simulink model "SolarSailOld"  (R2024a)
settings: Solver=VariableStepAuto  StartTime=0.0  StopTime=60*120  RelTol=1e-3
model workspace (MAT data in the model file):
  LocalBodyOffset = [45 0 0]
undefined symbols (not defined in the file): juliandate, magnitude
libraries: aerolibutil x12, matrix_library x8, aerolibconvert2 x4, sharedtransform x4, slpidlib x2, simulink_extras x2, aerolibsatdyn x1, aerolibobsolete x1, aerolibattitudesys x1, simulink x1, vrlib x1
(part 1 of 2)
settings Model: Creator=pierc  LastModifiedBy=Spare

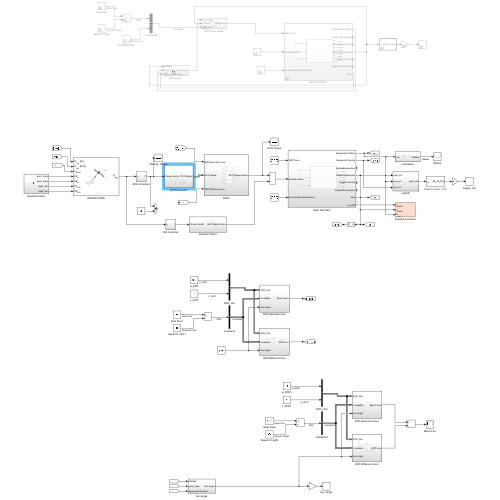
[thumbnail: Simulink's stored preview of the top-level diagram]
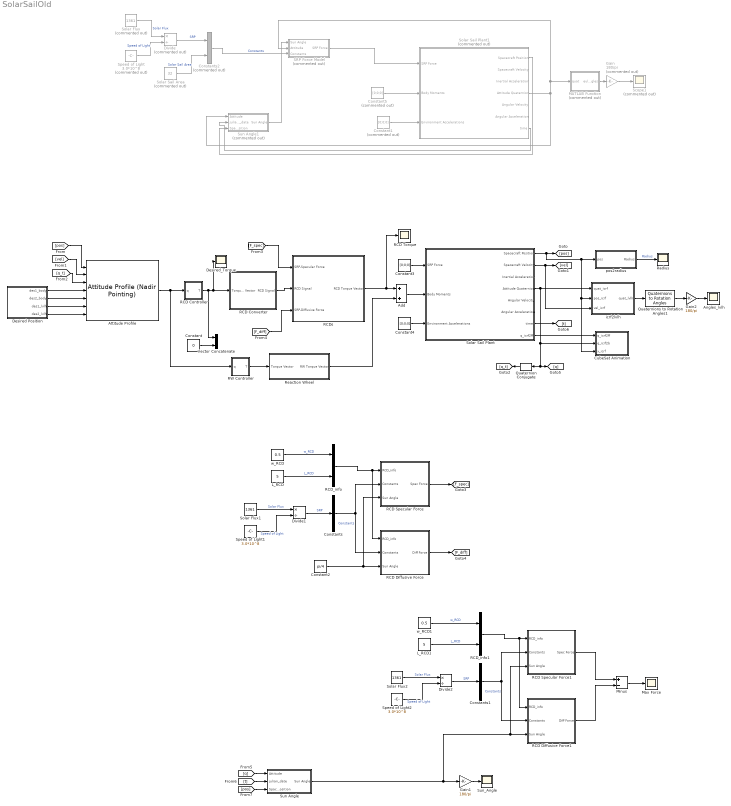
== system SolarSailOld ==
  Add : Sum
  Angles_lvlh : Scope
  "Attitude Profile " : aerolibsatdyn/Attitude Profile (Nadir Pointing)  outputError=on  outputFinalAttitude=off  portFrame=ICRF  pointingMode=Custom  celestialTarget=Sun  tunablePointing=off  primaryAlignmentSrc=Port  primaryAlignment=[0 0 1]  secondaryAlignmentSrc=Port  secondaryAlignment=[1 0 0]  constraintFrame=LVLH  primaryConstraintSrc=Port  primaryConstraint=[1 0 0]  secondaryConstraintSrc=Port  secondaryConstraint=[0 1 0]
  Constant : Constant  Value=0
  Constant1 : Constant  Commented=on  Value=[0;0;0]
  Constant2 : Constant  Value=pi/4
  Constant3 : Constant  Value=[0;0;0]
  Constant4 : Constant  Value=[0;0;0]
  Constant5 : Constant  Commented=on  Value=[0;0;0]
  Constants : BusCreator  Inputs=1
  Constants1 : BusCreator  Inputs=1
  Constants2 : BusCreator  Commented=on  Inputs=2
  CubeSat Animation : Subsystem  mask(Simulink 3D Animation of CubeSat){enableVis=on, startDate=juliandate(2024, 7, 11, 2, 0, 0), visSampleTime=10, cubesatSize=2e5, showAntenna=on, antennaHeight=1e6, antennaHalfAngle=15}
      mask prompts: enableVis "spacecraft:cubesat:AnimEnableVis"; startDate "spacecraft:cubesat:StartDate"; visSampleTime "spacecraft:cubesat:AnimSampleTime"; cubesatSize "spacecraft:cubesat:MdlSize"; showAntenna "spacecraft:cubesat:ShowCone"; antennaHeight "spacecraft:cubesat:ConeHeight"; antennaHalfAngle "spacecraft:cubesat:ConeAngle"
      mask help: spacecraft:cubesat:VisBlockDesc
      settings: OpenFcn=|
      | if ~builtin('license','test','virtual_reality_toolbox')
      |     set_param(gcb, 'enableVis', 'off');
      | end
      | open_system(gcb,'mask');
      mask Callback enableVis:
      | if strcmp(get_param(gcb,'enableVis'), 'on')
      |     [licAvail, ~] = builtin('license','checkout','Virtual_Reality_Toolbox');
      |     if licAvail
      |         enable = repmat({'on'},7,1);
      |         set_param(gcb, 'Commented', 'off');
      |     else
      |         enable = repmat({'off'},7,1);
      |         set_param(gcb, 'Commented', 'on');
      |         set_param(gcb,'enableVis', 'off');
      |     end
      |     clear licAvail
      | else
      |     enable = repmat({'off'},7,1);
      |     set_param(gcb, 'Commented', 'on');
      | end
      | enable{1} = 'on';
      | set_param(gcb,'MaskEnables', enable);
      | clear enable
      mask Callback showAntenna:
      | if strcmp(get_param(gcb, 'enableVis'), 'on')
      |     enable = get_param(gcb,'MaskEnables');
      |     if strcmp(get_param(gcb, 'showAntenna'), 'off')
      |         enable(6:7) = {'off'};
      |     else
      |         enable(6:7) = {'on'};
      |     end
      |     set_param(gcb,'MaskEnables', enable);
      |     clear enable
      | end
      mask DialogControl enableVis Prompt: Enable visualization with Simulink 3D Animation
      mask DialogControl vrOpenBtn Prompt: spacecraft:cubesat:AnimOpenBtn
      mask DialogControl vrOpenBtn Callback:
      | if builtin('license','checkout','Virtual_Reality_Toolbox')
      |     vrmfunc('FnOpen',getSimulinkBlockHandle([gcb '/VR Sink']));
      | end
      mask DialogControl startDate Prompt: Start date [Julian date]:
      mask DialogControl startDate Tooltip: spacecraft:cubesat:StartDateTT
      mask DialogControl visSampleTime Prompt: Animation refresh rate:
      mask DialogControl visSampleTime Tooltip: spacecraft:cubesat:AnimSampleTimeTT
      mask DialogControl cubesatSize Prompt: CubeSat display size [m]:
      mask DialogControl cubesatSize Tooltip: spacecraft:cubesat:MdlSizeTT
      mask DialogControl Container3 Prompt: spacecraft:cubesat:AntennaPropArea
      mask DialogControl showAntenna Prompt: Show antenna cone in animation
      mask DialogControl showAntenna Tooltip: spacecraft:cubesat:ShowConeTT
      mask DialogControl antennaHeight Prompt: Antenna cone height [m]:
      mask DialogControl antennaHeight Tooltip: spacecraft:cubesat:ConeHeightTT
      mask DialogControl antennaHalfAngle Prompt: Antenna cone half angle [deg]:
      mask DialogControl antennaHalfAngle Tooltip: spacecraft:cubesat:ConeAngleTT
      mask Display:
      | port_label('input', 3, 'X_{icrf}','texmode','on')
      | port_label('input', 2, 'q_{icrf2b}','texmode','on')
      | port_label('input', 1, 'q_{icrf2ff}','texmode','on')
  Desired Position : Subsystem
  Desired_Torque : Scope
  Divide : Product  Commented=on  Inputs=*/
  Divide1 : Product  Inputs=*/
  Divide2 : Product  Inputs=*/
  Gain : Gain  Commented=on  Gain=180/pi
  Gain1 : Gain  Gain=180/pi
  Gain2 : Gain  Gain=180/pi
  L_RCD : Constant  Value=5
  L_RCD1 : Constant  Value=5
  MATLAB Function : MATLAB Function  Commented=on  TreatAsAtomicUnit=on
  Max Force : Scope
  Minus : Sum  Inputs=+-
  Quaternion Conjugate : aerolibutil/Quaternion Conjugate
  Quaternions to Rotation Angles1 : sharedtransform/Quaternions to Rotation Angles  rotationOrder=ZYX  aMode=aMode
  RCD Controller : Subsystem
  RCD Converter : Subsystem
  RCD Diffusive Force : Subsystem
  RCD Diffusive Force1 : Subsystem
  RCD Specular Force : Subsystem
  RCD Specular Force1 : Subsystem
  RCD Torque : Scope
  RCD_info : BusCreator  Inputs=2
  RCD_info1 : BusCreator  Inputs=2
  RCDs : Subsystem
  RW Controller : Subsystem
  Radius : Scope
  Reaction Wheel : Subsystem
  SRP Force Model : Subsystem  Commented=on
  Scope1 : Scope  Commented=on
  Solar Flux : Constant  Commented=on  Value=1361
  Solar Flux1 : Constant  Value=1361
  Solar Flux2 : Constant  Value=1361
  Solar Sail Area : Constant  Commented=on  Value=32
  Solar Sail Plant : Subsystem
  Solar Sail Plant1 : Subsystem  Commented=on
  Speed of Light : Constant  Commented=on  Value=3.0*10^8
  Speed of Light1 : Constant  Value=3.0*10^8
  Speed of Light2 : Constant  Value=3.0*10^8
  Sun Angle : Subsystem
  Sun Angle1 : Subsystem  Commented=on
  Sun_Angle : Scope
  Vector Concatenate : Concatenate
  icrf2lvlh : Subsystem
  pos2radius : Subsystem
  w_RCD : Constant  Value=0.5
  w_RCD1 : Constant  Value=0.5
  wires:
  SRP Force Model/1(SRP Force) -> Solar Sail Plant1/1(SRP Force)
  Solar Sail Area/1 -> Constants2/2  "Solar Sail Area"
  Constants2/1 -> SRP Force Model/3(Constants)  "Constants"
  Sun Angle1/1(Sun Angle) -> SRP Force Model/1(Sun Angle)
  Solar Sail Plant1/7(time) -> Sun Angle1/2(julian_date)
  Solar Sail Plant1/1(Spacecraft Position) -> Sun Angle1/3(Spacecraft Position)
  Solar Sail Plant1/4(Attitude Quaternion) -> Sun Angle1/1(Attitude), MATLAB Function/1(quat), SRP Force Model/2(Attitude)
  Constant5/1 -> Solar Sail Plant1/2(Body Moments)
  Constant1/1 -> Solar Sail Plant1/3(Environment Accelerations)
  MATLAB Function/1(eulerAngles) -> Gain/1
  Gain/1 -> Scope1/1
  Solar Sail Plant/1(Spacecraft Position) -> icrf2lvlh/2(pos_icrf), CubeSat Animation/3(x_icrf), pos2radius/1(pos), [pos]
  Solar Sail Plant/4(Attitude Quaternion) -> Quaternion Conjugate/1, [q], CubeSat Animation/2(q_icrf2b), icrf2lvlh/1(quat_icrf)
  Constant3/1 -> Solar Sail Plant/1(SRP Force)
  Constant4/1 -> Solar Sail Plant/3(Environment Accelerations)
  pos2radius/1(Radius) -> Radius/1  "Radius"
  Solar Sail Plant/8(q_icrf2ff) -> CubeSat Animation/1(q_icrf2ff)
  Gain2/1 -> Angles_lvlh/1
  L_RCD/1 -> RCD_info/2  "L_RCD"
  RCD_info/1 -> RCD Diffusive Force/1(RCD_info), RCD Specular Force/1(RCD_info)
  Solar Flux/1 -> Divide/1  "Solar Flux"
  Speed of Light/1 -> Divide/2  "Speed of Light"
  Divide/1 -> Constants2/1  "SRP"
  RCD Controller/1(T) -> Vector Concatenate/1, Desired_Torque/1, RCD Converter/1(Torque Vector)
  [pos] -> "Attitude Profile "/1
  Solar Sail Plant/2(Spacecraft Velocity) -> [vel], icrf2lvlh/3(vel_icrf)
  [vel] -> "Attitude Profile "/2
  Quaternion Conjugate/1 -> [q_t]
  [q_t] -> "Attitude Profile "/3
  Constants/1 -> RCD Specular Force/2(Constants), RCD Diffusive Force/2(Constants)  "Constants"
  Solar Flux1/1 -> Divide1/1  "Solar Flux"
  Speed of Light1/1 -> Divide1/2  "Speed of Light"
  Divide1/1 -> Constants/1  "SRP"
  [F_spec] -> RCDs/1(SRP-Specular Force)
  RCDs/1(RCD Torque Vector) -> Add/1, RCD Torque/1
  RCD Converter/1(RCD Signal) -> RCDs/2(RCD Signal)
  Reaction Wheel/1(RW Torque Vector) -> Add/2
  icrf2lvlh/1(quat_lvlh) -> Quaternions to Rotation Angles1/1
  Quaternions to Rotation Angles1/1 -> Gain2/1
  Desired Position/3(des1_lvlh) -> "Attitude Profile "/6
  Desired Position/4(des2_lvlh) -> "Attitude Profile "/7
  w_RCD/1 -> RCD_info/1  "w_RCD"
  RCD Specular Force/1(Spec Force) -> [F_spec]
  RCD Diffusive Force/1(Diff Force) -> [F_diff]
  [F_diff] -> RCDs/3(SRP-Diffusive Force)
  "Attitude Profile "/1 -> RW Controller/1(q), RCD Controller/1(q)
  Desired Position/1(des1_body) -> "Attitude Profile "/4
  Desired Position/2(des2_body) -> "Attitude Profile "/5
  Add/1 -> Solar Sail Plant/2(Body Moments)
  RW Controller/1(T) -> Reaction Wheel/1(Torque Vector)
  Solar Sail Plant/7(time) -> [t]
  [t] -> Sun Angle/2(julian_date)
  [q] -> Sun Angle/1(Attitude)
  [pos] -> Sun Angle/3(Spacecraft Position)
  Gain1/1 -> Sun_Angle/1
  Constant/1 -> Vector Concatenate/2
  Speed of Light2/1 -> Divide2/2  "Speed of Light"
  w_RCD1/1 -> RCD_info1/1  "w_RCD"
  RCD Specular Force1/1(Spec Force) -> Minus/1
  RCD Diffusive Force1/1(Diff Force) -> Minus/2
  RCD_info1/1 -> RCD Diffusive Force1/1(RCD_info), RCD Specular Force1/1(RCD_info)
  Divide2/1 -> Constants1/1  "SRP"
  Solar Flux2/1 -> Divide2/1  "Solar Flux"
  Constants1/1 -> RCD Specular Force1/2(Constants), RCD Diffusive Force1/2(Constants)  "Constants"
  Sun Angle/1(Sun Angle) -> RCD Specular Force1/3(Sun Angle), RCD Diffusive Force1/3(Sun Angle), Gain1/1
  L_RCD1/1 -> RCD_info1/2  "L_RCD"
  Minus/1 -> Max Force/1
  Constant2/1 -> RCD Specular Force/3(Sun Angle), RCD Diffusive Force/3(Sun Angle)

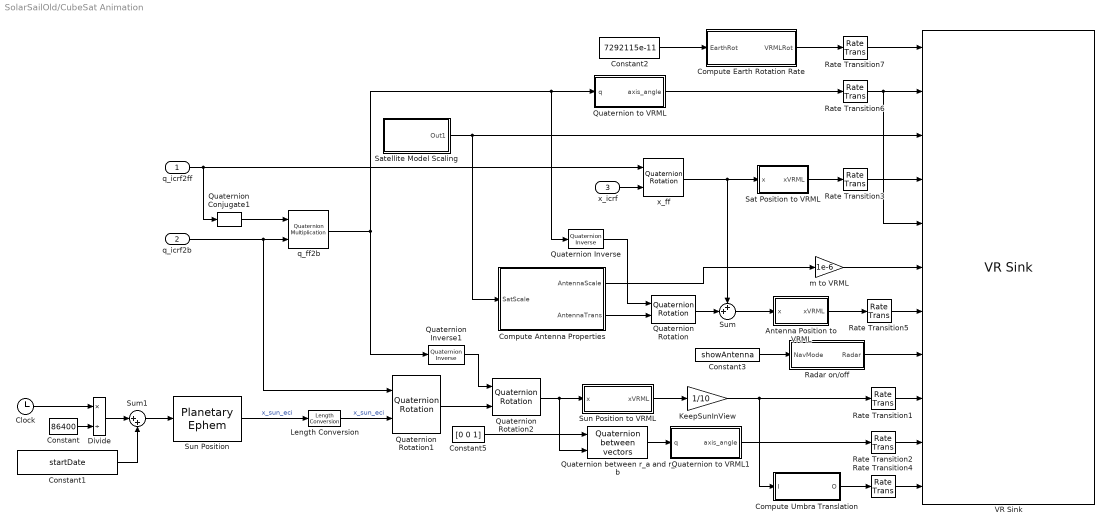
== system SolarSailOld/CubeSat Animation ==
  q_icrf2ff : Inport  PortDimensions=4
  q_icrf2b : Inport  Port=2  PortDimensions=4
  x_icrf : Inport  Port=3  PortDimensions=3
  Antenna Position to VRML : Subsystem
  Clock : Clock
  Compute Antenna Properties : Subsystem
  Compute Earth Rotation Rate : Subsystem
  Compute Umbra Translation : Subsystem
  Constant : Constant  Value=86400
  Constant1 : Constant  Value=startDate  SampleTime=visSampleTime
  Constant2 : Constant  Value=7292115e-11
  Constant3 : Constant  Value=showAntenna
  Constant5 : Constant  Value=[0 0 1]
  Divide : Product  Inputs=*/
  KeepSunInView : Gain  Gain=1/10
  Length Conversion : aerolibconvert2/Length Conversion  IU=km  OU=m
  Quaternion Conjugate1 : aerolibutil/Quaternion Conjugate
  Quaternion Inverse : aerolibutil/Quaternion Inverse
  Quaternion Inverse1 : aerolibutil/Quaternion Inverse
  Quaternion Rotation : aerolibutil/Quaternion Rotation
  Quaternion Rotation1 : aerolibutil/Quaternion Rotation
  Quaternion Rotation2 : aerolibutil/Quaternion Rotation
  Quaternion between r_a and r_b : aerolibattitudesys/Quaternion between vectors
  Quaternion to VRML : Subsystem
  Quaternion to VRML1 : Subsystem
  Radar on/off : Subsystem
  Rate Transition{1..7} (7 alike) : RateTransition
  Sat Position to VRML : Subsystem
  Satellite Model Scaling : Subsystem
  Sum : Sum  Inputs=++|
  Sum1 : Sum  Inputs=|++
  Sun Position : PlanetaryEphem  ephemerisModel=DE421  target=Sun  outputVelocity=off
  Sun Position to VRML : Subsystem
  VR Sink : vrlib/VR Sink  InstantiateOnLoad=on  SampleTime=visSampleTime  ViewEnable=on  RemoteChange=off  RemoteView=off  FieldsWritten=Earth.rotation.4.1.1.double#Satellite.rotation.4.1.1.double#Satellite.scale.3.1.1.double#Satellite.translation.3.1.1.double#AntennaCone.rotation.4.1.1.double#AntennaCone.scale.3.1.1.double#AntennaCone.translation.3.1.1.double#AntennaMaterial.transparency.1.1.1.double#Sun.translation.3.1.1.double#Umbra.rotation.4.1.1.double#Umbra.translation.3.1.1.double  WorldFileName=cubesatAnim.wrl  WorldDescription=CubeSat Orbit Animation  AutoView=off  VideoDimensions=[]  AllowVariableSize=off  FigureProperties="{'Position', 'Name', 'Viewpoint', 'CameraBound', 'CameraDirection', 'CameraPosition', 'CameraUpVector', 'ZoomFactor', 'Antialiasing', 'Headlight', 'Lighting', 'Sound', 'StatusBar', 'Stereo3D', 'Stereo3DCameraOffset', 'Stereo3DHIT', 'ToolBar', 'Textures', 'Transparency', 'Triad', 'Wireframe', 'NavZones', 'NavMode', 'NavSpeed', 'CaptureFileFormat', 'CaptureFileName', 'Record2DCompressMethod', 'Record2DCompressQuality', 'Record2D', 'Record2DFileName', 'Record2DFPS', 'NavPanel'; [1.0000000000000000e+00   7.6000000000000000e+01   1.9200000000000000e+03   9.1300000000000000e+02], 'CubeSat Orbit Animation', 'Satellite-fixed', 'on', [1.8532076975005182e-02   1.5658460164834759e-01  -9.8750612734233556e-01], [5.1717154537575027e-02  -2.3230877286223661e+00  -8.9856200709735745e-01], [-6.2587088021580528e-02   9.8591804959445684e-01   1.5515964991196535e-01], [1.0000000000000000e+00], 'on', 'on', 'on', 'on', 'on', 'off', [1.0000000149011612e-01], [0.0000000000000000e+00], 'on', 'on', 'on', 'none', 'off', 'off', 'examine', 'normal', 'tif', '%f_anim_%n.tif', 'auto', [7.5000000000000000e+01], 'off', '%f_anim_%n.avi', 'auto', 'halfbar'}"
  m to VRML : Gain  Gain=1e-6
  q_ff2b : aerolibutil/Quaternion Multiplication
  x_ff : aerolibutil/Quaternion Rotation
  wires:
  Quaternion to VRML1/1(axis_angle) -> Rate Transition2/1
  Quaternion between r_a and r_b/1 -> Quaternion to VRML1/1(q)
  Constant2/1 -> Compute Earth Rotation Rate/1(EarthRot)
  Compute Antenna Properties/1(AntennaScale) -> m to VRML/1
  Quaternion to VRML/1(axis_angle) -> Rate Transition6/1
  Compute Umbra Translation/1(O) -> Rate Transition4/1
  q_icrf2b/1 -> Quaternion Rotation1/1, q_ff2b/2
  Quaternion Rotation2/1 -> Sun Position to VRML/1(x), Quaternion between r_a and r_b/2
  Constant5/1 -> Quaternion between r_a and r_b/1
  KeepSunInView/1 -> Compute Umbra Translation/1(I), Rate Transition1/1
  Sun Position to VRML/1(xVRML) -> KeepSunInView/1
  Sat Position to VRML/1(xVRML) -> Rate Transition3/1
  Compute Antenna Properties/2(AntennaTrans) -> Quaternion Rotation/2
  Satellite Model Scaling/1(Out1) -> VR Sink/3, Compute Antenna Properties/1(SatScale)
  Constant3/1 -> Radar on/off/1(NavMode)
  q_ff2b/1 -> Quaternion Inverse/1, Quaternion to VRML/1(q), Quaternion Inverse1/1
  Quaternion Rotation1/1 -> Quaternion Rotation2/2
  Compute Earth Rotation Rate/1(VRMLRot) -> Rate Transition7/1
  Antenna Position to VRML/1(xVRML) -> Rate Transition5/1
  Quaternion Inverse/1 -> Quaternion Rotation/1
  x_ff/1 -> Sum/1, Sat Position to VRML/1(x)
  Quaternion Rotation/1 -> Sum/2
  Sum/1 -> Antenna Position to VRML/1(x)
  Quaternion Inverse1/1 -> Quaternion Rotation2/1
  Rate Transition4/1 -> VR Sink/11
  Rate Transition2/1 -> VR Sink/10
  Rate Transition1/1 -> VR Sink/9
  Rate Transition5/1 -> VR Sink/7
  m to VRML/1 -> VR Sink/6
  Rate Transition3/1 -> VR Sink/4
  Rate Transition7/1 -> VR Sink/1
  Rate Transition6/1 -> VR Sink/5, VR Sink/2
  Constant1/1 -> Sum1/2
  Divide/1 -> Sum1/1
  Constant/1 -> Divide/2
  Sun Position/1 -> Length Conversion/1  "x_sun_eci"
  Clock/1 -> Divide/1
  Length Conversion/1 -> Quaternion Rotation1/2  "x_sun_eci"
  Sum1/1 -> Sun Position/1
  Radar on/off/1(Radar) -> VR Sink/8
  Quaternion Conjugate1/1 -> q_ff2b/1
  q_icrf2ff/1 -> Quaternion Conjugate1/1, x_ff/1
  x_icrf/1 -> x_ff/2

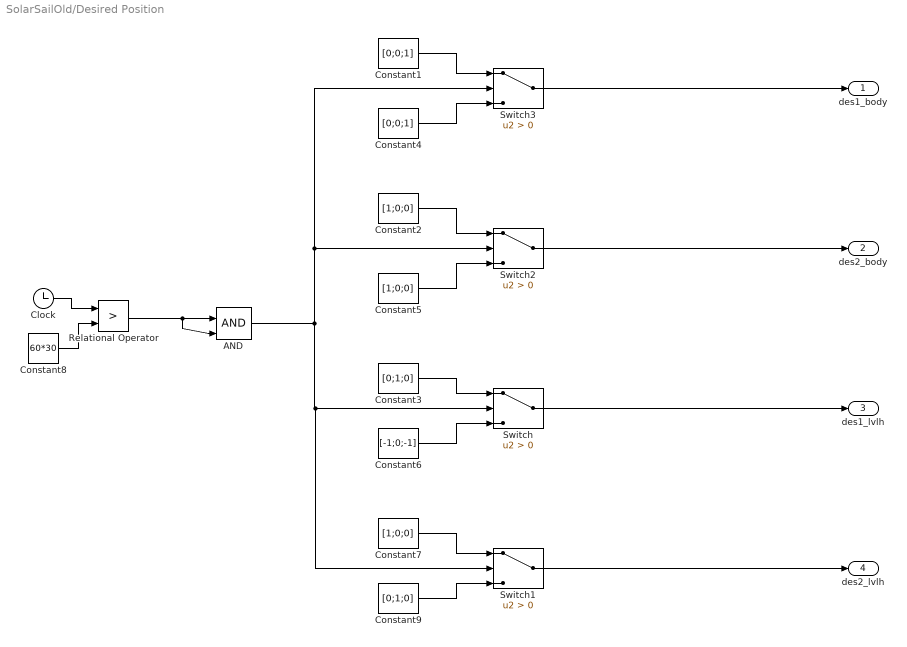
== system SolarSailOld/Desired Position ==
  AND : Logic  IconShape=distinctive  AllPortsSameDT=off  OutDataTypeStr=boolean
  Clock : Clock
  Constant1 : Constant  Value=[0;0;1]
  Constant2 : Constant  Value=[1;0;0]
  Constant3 : Constant  Value=[0;1;0]
  Constant4 : Constant  Value=[0;0;1]
  Constant5 : Constant  Value=[1;0;0]
  Constant6 : Constant  Value=[-1;0;-1]
  Constant7 : Constant  Value=[1;0;0]
  Constant8 : Constant  Value=60*30
  Constant9 : Constant  Value=[0;1;0]
  Relational Operator : RelationalOperator  Operator=>  OutDataTypeStr=boolean  RndMeth=Simplest  InputSameDT=off
  Switch{,1..3} (4 alike) : Switch  Criteria=u2 > Threshold  SaturateOnIntegerOverflow=off  InputSameDT=off
  des1_body : Outport
  des2_body : Outport  Port=2
  des1_lvlh : Outport  Port=3
  des2_lvlh : Outport  Port=4
  wires:
  Constant8/1 -> Relational Operator/2
  Constant6/1 -> Switch/3
  Clock/1 -> Relational Operator/1
  Constant9/1 -> Switch1/3
  Constant4/1 -> Switch3/3
  Constant5/1 -> Switch2/3
  Switch3/1 -> des1_body/1
  Switch2/1 -> des2_body/1
  Switch/1 -> des1_lvlh/1
  Switch1/1 -> des2_lvlh/1
  Constant1/1 -> Switch3/1
  Constant2/1 -> Switch2/1
  Constant7/1 -> Switch1/1
  Constant3/1 -> Switch/1
  AND/1 -> Switch1/2, Switch/2, Switch3/2, Switch2/2
  Relational Operator/1 -> AND/2, AND/1

== system SolarSailOld/RCD Controller ==
  q : Inport
  Demo Controller : slpidlib/PID Controller  Controller=PID  Form=Parallel  TimeDomain=Discrete-time  UseExternalTs=off  SampleTime=-1  IntegratorMethod=Trapezoidal  FilterMethod=Trapezoidal  ControllerParametersSource=internal  P=.0000022  I=0  UseKiTs=off  D=.0015  UseExternalDerivativeSource=off  N=1  UseFilter=off  TunerSelectOption=Transfer Function Based (PID Tuner App)  InitialConditionSource=internal  InitialConditionForIntegrator=0  InitialConditionForFilter=0  DifferentiatorICPrevScaledInput=0  ExternalReset=none  TrackingMode=off  Kt=1  LimitOutput=on  SatLimitsSource=internal  UpperSaturationLimit=0.008  LowerSaturationLimit=-0.008  LinearizeAsGain=on  AntiWindupMode=none  Kb=1  LimitIntegrator=off  UpperIntegratorSaturationLimit=inf  LowerIntegratorSaturationLimit=-inf  POutMin=[]  POutMax=[]  IOutMin=[]  IOutMax=[]  DOutMin=[]  DOutMax=[]  NOutMin=[]  NOutMax=[]  SumOutMin=[]  SumOutMax=[]  SaturationOutMin=[]  SaturationOutMax=[]  PParamMin=[]  PParamMax=[]  IParamMin=[]  IParamMax=[]  DParamMin=[]  DParamMax=[]  NParamMin=[]  NParamMax=[]  KbParamMin=[]  KbParamMax=[]  KtParamMin=[]  KtParamMax=[]  KbOutMin=[]  KbOutMax=[]  KtOutMin=[]  KtOutMax=[]  IntegratorOutMin=[]  IntegratorOutMax=[]  FilterOutMin=[]  FilterOutMax=[]  SumI1OutMin=[]  SumI1OutMax=[]  SumI2OutMin=[]  SumI2OutMax=[]  SumI3OutMin=[]  SumI3OutMax=[]  SumI4OutMin=[]  SumI4OutMax=[]  SumDOutMin=[]  SumDOutMax=[]  DifferentiatorOutMin=[]  DifferentiatorOutMax=[]  FilterDiffOutCoefMin=[]  FilterDiffOutCoefMax=[]  ReciprocalOutMin=[]  ReciprocalOutMax=[]  SumDenOutMin=[]  SumDenOutMax=[]  SumNumOutMin=[]  SumNumOutMax=[]  DivideOutMin=[]  DivideOutMax=[]  UdiffTsProdOutMin=[]  UdiffTsProdOutMax=[]  NTsProdOutMin=[]  NTsProdOutMax=[]  UintegralTsProdOutMin=[]  UintegralTsProdOutMax=[]  UngainTsProdOutMin=[]  UngainTsProdOutMax=[]  ClampingZeroOutDataTypeStr=Inherit: Inherit via back propagation  ClampingZeroOutMin=[]  ClampingZeroOutMax=[]  FilterDenConstantOutDataTypeStr=Inherit: Inherit via back propagation  FilterDenConstantOutMin=[]  FilterDenConstantOutMax=[]  PCopyOutDataTypeStr=Inherit: Inherit via back propagation  PCopyOutMin=[]  PCopyOutMax=[]  NCopyOutDataTypeStr=Inherit: Inherit via back propagation  NCopyOutMin=[]  NCopyOutMax=[]  IntegratorContinuousStateAttributes=''  IntegratorStateMustResolveToSignalObject=off  IntegratorRTWStateStorageClass=Auto  FilterContinuousStateAttributes=''  FilterStateMustResolveToSignalObject=off  FilterRTWStateStorageClass=Auto  ParallelPVariant=InternalParameters  IdealPVariant=Disabled  IVariant=InternalParameters  DVariant=InternalParameters  IntegratorVariant=Discrete  SatVariant=Enabled  AWVariant=Passthrough  PCopyVariant=Disabled  TRVariant=Disabled  FdbkBlocksVariant=Forward  IdealPFdbkVariant=Disabled  SatFdbkVariant=Disabled  DerivativeFilterVariant=Differentiator  NVariant=Passthrough  NCopyVariant=Disabled_SignalSpec  FilterICVariant=InternalICsDifferentiator  IntegratorICVariant=InternalICs  ExternalResetVariant=Disabled  TRSumVariant=Passthrough  SumFdbkVariant=Disabled  SumVariant=Sum_PID  TsampFilterVariant=InternalTs  TsampNgainVariant=Passthrough  TsampIntegralVariant=Disabled_SignalSpec  ExternalSaturationOutDataTypeStr=Inherit: Same as second input  DerivativeSourceVariant=ErrorSignal
  Quaternions to Rotation Angles : sharedtransform/Quaternions to Rotation Angles  rotationOrder=XYZ  aMode=aMode
  Selector : Selector  InputPortWidth=3  IndexOptions=Index vector (dialog)  Indices=[1;2]  OutputSizes=1
  T : Outport
  wires:
  q/1 -> Quaternions to Rotation Angles/1
  Demo Controller/1 -> T/1
  Selector/1 -> Demo Controller/1
  Quaternions to Rotation Angles/1 -> Selector/1

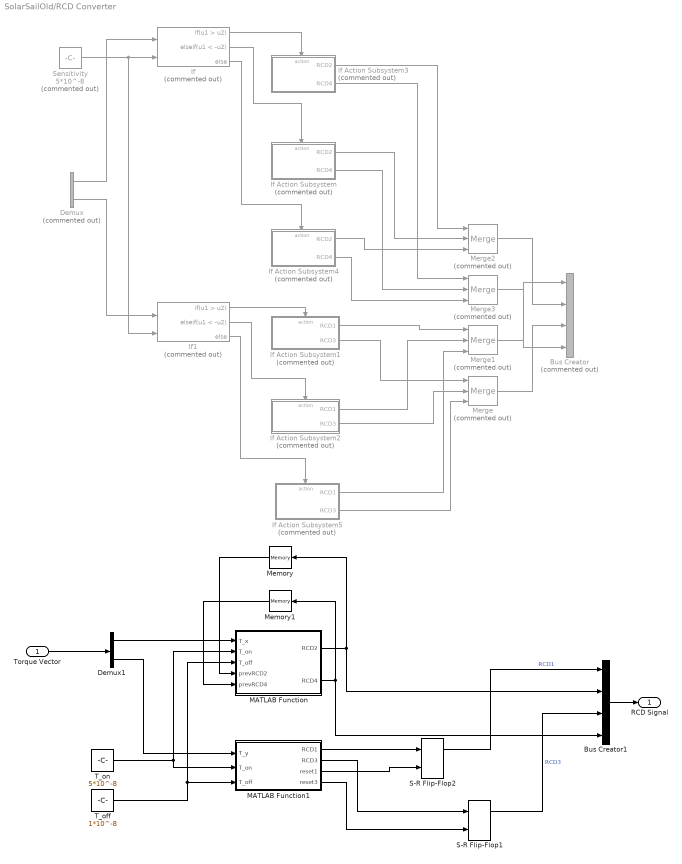
== system SolarSailOld/RCD Converter ==
  Torque Vector : Inport
  Bus Creator : BusCreator  Commented=on  Inputs=4
  Bus Creator1 : BusCreator  Inputs=4
  Demux : Demux  Commented=on  Outputs=2
  Demux1 : Demux  Outputs=2
  If : If  Commented=on  NumInputs=2  IfExpression=u1 > u2  ElseIfExpressions=u1 < -u2
  If Action Subsystem : Subsystem  Commented=on  TreatAsAtomicUnit=on
  If Action Subsystem1 : Subsystem  Commented=on  TreatAsAtomicUnit=on
  If Action Subsystem2 : Subsystem  Commented=on  TreatAsAtomicUnit=on
  If Action Subsystem3 : Subsystem  Commented=on  TreatAsAtomicUnit=on
  If Action Subsystem4 : Subsystem  Commented=on  TreatAsAtomicUnit=on
  If Action Subsystem5 : Subsystem  Commented=on  TreatAsAtomicUnit=on
  If1 : If  Commented=on  NumInputs=2  IfExpression=u1 > u2  ElseIfExpressions=u1 < -u2
  MATLAB Function : MATLAB Function  TreatAsAtomicUnit=on
  MATLAB Function1 : MATLAB Function  TreatAsAtomicUnit=on
  Memory : Memory
  Memory1 : Memory
  Merge{,1..3} (4 alike) : Merge  Commented=on  Inputs=3
  S-R Flip-Flop1 : simulink_extras/Flip Flops/S-R Flip-Flop  initial_condition=0
  S-R Flip-Flop2 : simulink_extras/Flip Flops/S-R Flip-Flop  initial_condition=0
  Sensitivity : Constant  Commented=on  Value=5*10^-8
  T_off : Constant  Value=1*10^-8
  T_on : Constant  Value=5*10^-8
  RCD Signal : Outport
  wires:
  If/1 -> If Action Subsystem3/Action
  If1/1 -> If Action Subsystem1/Action
  If/2 -> If Action Subsystem/Action
  Demux/2 -> If1/1
  Demux/1 -> If/1
  If1/2 -> If Action Subsystem2/Action
  If Action Subsystem1/2(RCD3) -> Merge/1
  Merge/1 -> Bus Creator/3
  If Action Subsystem2/2(RCD3) -> Merge/2
  If Action Subsystem1/1(RCD1) -> Merge1/1
  If Action Subsystem2/1(RCD1) -> Merge1/2
  Merge1/1 -> Bus Creator/1
  Merge2/1 -> Bus Creator/2
  Merge3/1 -> Bus Creator/4
  If Action Subsystem/2(RCD4) -> Merge3/2
  If Action Subsystem/1(RCD2) -> Merge2/2
  If Action Subsystem3/2(RCD4) -> Merge3/1
  If Action Subsystem3/1(RCD2) -> Merge2/1
  Sensitivity/1 -> If/2, If1/2
  If/3 -> If Action Subsystem4/Action
  If Action Subsystem4/2(RCD4) -> Merge3/3
  If Action Subsystem4/1(RCD2) -> Merge2/3
  If1/3 -> If Action Subsystem5/Action
  If Action Subsystem5/1(RCD1) -> Merge1/3
  If Action Subsystem5/2(RCD3) -> Merge/3
  T_on/1 -> MATLAB Function/2(T_on), MATLAB Function1/2(T_on)
  T_off/1 -> MATLAB Function/3(T_off), MATLAB Function1/3(T_off)
  Torque Vector/1 -> Demux1/1
  Demux1/1 -> MATLAB Function/1(T_x)
  Demux1/2 -> MATLAB Function1/1(T_y)
  Bus Creator1/1 -> RCD Signal/1
  MATLAB Function/1(RCD2) -> Memory/1, Bus Creator1/2
  MATLAB Function/2(RCD4) -> Memory1/1, Bus Creator1/4
  Memory/1 -> MATLAB Function/4(prevRCD2)
  Memory1/1 -> MATLAB Function/5(prevRCD4)
  MATLAB Function1/1(RCD1) -> S-R Flip-Flop2/1
  MATLAB Function1/3(reset1) -> S-R Flip-Flop2/2
  MATLAB Function1/2(RCD3) -> S-R Flip-Flop1/1
  MATLAB Function1/4(reset3) -> S-R Flip-Flop1/2
  S-R Flip-Flop1/1 -> Bus Creator1/3  "RCD3"
  S-R Flip-Flop2/1 -> Bus Creator1/1  "RCD1"

== system SolarSailOld/RCD Diffusive Force ==
  Bus Element In : Inport  PortName=RCD_info  Element=w_RCD
  BusElementIn1 : Inport  PortName=RCD_info  Element=L_RCD
  Bus Element In1 : Inport  Port=2  PortName=Constants  Element=SRP
  Sun Angle : Inport  Port=3
  Add : Sum
  Cos : Trigonometry  Operator=cos
  F_normal : Subsystem
  F_sun : Subsystem
  Product : Product
  Product1 : Product
  Diff Force : Outport
  wires:
  BusElementIn1/1 -> Product/1
  Bus Element In/1 -> Product/2
  Sun Angle/1 -> Cos/1, F_sun/3(sun anlge), F_normal/3(sun anlge)
  Bus Element In1/1 -> F_sun/1(SRP), F_normal/1(SRP)
  Product/1 -> F_sun/2(area), F_normal/2(area)  "area"
  F_sun/1(F_sun) -> Product1/1
  Cos/1 -> Product1/2
  Add/1 -> Diff Force/1
  F_normal/1(F_normal) -> Add/1
  Product1/1 -> Add/2

== system SolarSailOld/RCD Diffusive Force1 ==
  Bus Element In : Inport  PortName=RCD_info  Element=w_RCD
  BusElementIn1 : Inport  PortName=RCD_info  Element=L_RCD
  Bus Element In1 : Inport  Port=2  PortName=Constants  Element=SRP
  Sun Angle : Inport  Port=3
  Add : Sum
  Cos : Trigonometry  Operator=cos
  F_normal : Subsystem
  F_sun : Subsystem
  Product : Product
  Product1 : Product
  Diff Force : Outport
  wires:
  BusElementIn1/1 -> Product/1
  Bus Element In/1 -> Product/2
  Sun Angle/1 -> Cos/1, F_sun/3(sun anlge), F_normal/3(sun anlge)
  Bus Element In1/1 -> F_sun/1(SRP), F_normal/1(SRP)
  Product/1 -> F_sun/2(area), F_normal/2(area)  "area"
  F_sun/1(F_sun) -> Product1/1
  Cos/1 -> Product1/2
  Add/1 -> Diff Force/1
  F_normal/1(F_normal) -> Add/1
  Product1/1 -> Add/2

== system SolarSailOld/RCD Specular Force ==
  Bus Element In : Inport  PortName=RCD_info  Element=w_RCD
  BusElementIn1 : Inport  PortName=RCD_info  Element=L_RCD
  Bus Element In1 : Inport  Port=2  PortName=Constants  Element=SRP
  Sun Angle : Inport  Port=3
  Cos : Trigonometry  Operator=cos
  Gain : Gain  Gain=2
  Product : Product
  Product1 : Product  Inputs=3
  Square : Math  Operator=square
  Spec Force : Outport
  wires:
  BusElementIn1/1 -> Product/1
  Bus Element In/1 -> Product/2
  Square/1 -> Product1/3
  Bus Element In1/1 -> Product1/1
  Gain/1 -> Spec Force/1
  Sun Angle/1 -> Cos/1
  Product1/1 -> Gain/1
  Cos/1 -> Square/1
  Product/1 -> Product1/2  "area"

== system SolarSailOld/RCD Specular Force1 ==
  Bus Element In : Inport  PortName=RCD_info  Element=w_RCD
  BusElementIn1 : Inport  PortName=RCD_info  Element=L_RCD
  Bus Element In1 : Inport  Port=2  PortName=Constants  Element=SRP
  Sun Angle : Inport  Port=3
  Cos : Trigonometry  Operator=cos
  Gain : Gain  Gain=2
  Product : Product
  Product1 : Product  Inputs=3
  Square : Math  Operator=square
  Spec Force : Outport
  wires:
  BusElementIn1/1 -> Product/1
  Bus Element In/1 -> Product/2
  Square/1 -> Product1/3
  Bus Element In1/1 -> Product1/1
  Gain/1 -> Spec Force/1
  Sun Angle/1 -> Cos/1
  Product1/1 -> Gain/1
  Cos/1 -> Square/1
  Product/1 -> Product1/2  "area"

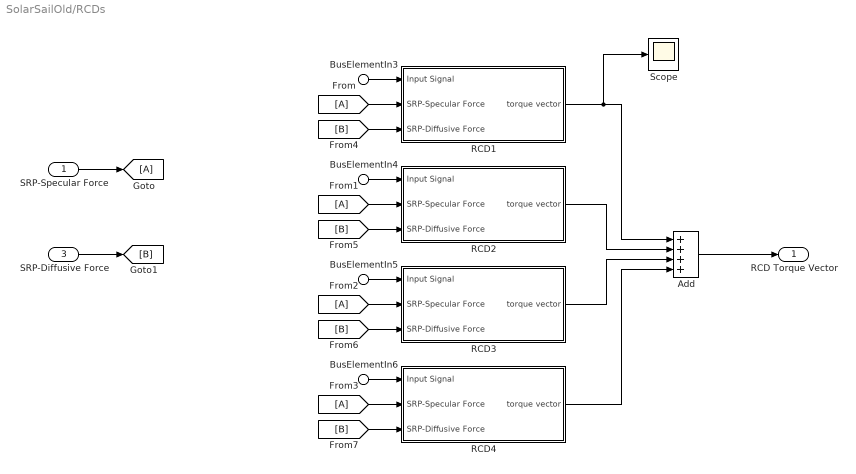
== system SolarSailOld/RCDs ==
  SRP-Specular Force : Inport
  BusElementIn3 : Inport  Port=2  PortName=RCD Signal  Element=RCD1
  BusElementIn4 : Inport  Port=2  PortName=RCD Signal  Element=RCD2
  BusElementIn5 : Inport  Port=2  PortName=RCD Signal  Element=RCD3
  BusElementIn6 : Inport  Port=2  PortName=RCD Signal  Element=RCD4
  SRP-Diffusive Force : Inport  Port=3
  Add : Sum  Inputs=++++
  From{,1..3} (4 alike) : From
  Goto : Goto
  RCD1 : Subsystem
  RCD2 : Subsystem
  RCD3 : Subsystem
  RCD4 : Subsystem
  Scope : Scope
  RCD Torque Vector : Outport
  wires:
  RCD2/1(torque vector) -> Add/2
  RCD1/1(torque vector) -> Scope/1, Add/1
  RCD4/1(torque vector) -> Add/4
  RCD3/1(torque vector) -> Add/3
  Add/1 -> RCD Torque Vector/1
  BusElementIn3/1 -> RCD1/1(Input Signal)
  BusElementIn4/1 -> RCD2/1(Input Signal)
  BusElementIn5/1 -> RCD3/1(Input Signal)
  SRP-Specular Force/1 -> Goto/1
  From/1 -> RCD1/2(SRP-Specular Force)
  From1/1 -> RCD2/2(SRP-Specular Force)
  From2/1 -> RCD3/2(SRP-Specular Force)
  From3/1 -> RCD4/2(SRP-Specular Force)
  [B] -> RCD1/3(SRP-Diffusive Force)
  [B] -> RCD2/3(SRP-Diffusive Force)
  [B] -> RCD3/3(SRP-Diffusive Force)
  [B] -> RCD4/3(SRP-Diffusive Force)
  SRP-Diffusive Force/1 -> [B]
  BusElementIn6/1 -> RCD4/1(Input Signal)

== system SolarSailOld/RW Controller ==
  q : Inport
  Demo Controller : slpidlib/PID Controller  Controller=PD  Form=Parallel  TimeDomain=Discrete-time  UseExternalTs=off  SampleTime=-1  IntegratorMethod=Trapezoidal  FilterMethod=Trapezoidal  ControllerParametersSource=internal  P=.000055  I=0  UseKiTs=off  D=.017  UseExternalDerivativeSource=off  N=1  UseFilter=off  TunerSelectOption=Transfer Function Based (PID Tuner App)  InitialConditionSource=internal  InitialConditionForIntegrator=0  InitialConditionForFilter=0  DifferentiatorICPrevScaledInput=0  ExternalReset=none  TrackingMode=off  Kt=1  LimitOutput=on  SatLimitsSource=internal  UpperSaturationLimit=0.008  LowerSaturationLimit=-0.008  LinearizeAsGain=on  AntiWindupMode=none  Kb=1  LimitIntegrator=off  UpperIntegratorSaturationLimit=inf  LowerIntegratorSaturationLimit=-inf  POutMin=[]  POutMax=[]  IOutMin=[]  IOutMax=[]  DOutMin=[]  DOutMax=[]  NOutMin=[]  NOutMax=[]  SumOutMin=[]  SumOutMax=[]  SaturationOutMin=[]  SaturationOutMax=[]  PParamMin=[]  PParamMax=[]  IParamMin=[]  IParamMax=[]  DParamMin=[]  DParamMax=[]  NParamMin=[]  NParamMax=[]  KbParamMin=[]  KbParamMax=[]  KtParamMin=[]  KtParamMax=[]  KbOutMin=[]  KbOutMax=[]  KtOutMin=[]  KtOutMax=[]  IntegratorOutMin=[]  IntegratorOutMax=[]  FilterOutMin=[]  FilterOutMax=[]  SumI1OutMin=[]  SumI1OutMax=[]  SumI2OutMin=[]  SumI2OutMax=[]  SumI3OutMin=[]  SumI3OutMax=[]  SumI4OutMin=[]  SumI4OutMax=[]  SumDOutMin=[]  SumDOutMax=[]  DifferentiatorOutMin=[]  DifferentiatorOutMax=[]  FilterDiffOutCoefMin=[]  FilterDiffOutCoefMax=[]  ReciprocalOutMin=[]  ReciprocalOutMax=[]  SumDenOutMin=[]  SumDenOutMax=[]  SumNumOutMin=[]  SumNumOutMax=[]  DivideOutMin=[]  DivideOutMax=[]  UdiffTsProdOutMin=[]  UdiffTsProdOutMax=[]  NTsProdOutMin=[]  NTsProdOutMax=[]  UintegralTsProdOutMin=[]  UintegralTsProdOutMax=[]  UngainTsProdOutMin=[]  UngainTsProdOutMax=[]  ClampingZeroOutDataTypeStr=Inherit: Inherit via back propagation  ClampingZeroOutMin=[]  ClampingZeroOutMax=[]  FilterDenConstantOutDataTypeStr=Inherit: Inherit via back propagation  FilterDenConstantOutMin=[]  FilterDenConstantOutMax=[]  PCopyOutDataTypeStr=Inherit: Inherit via back propagation  PCopyOutMin=[]  PCopyOutMax=[]  NCopyOutDataTypeStr=Inherit: Inherit via back propagation  NCopyOutMin=[]  NCopyOutMax=[]  IntegratorContinuousStateAttributes=''  IntegratorStateMustResolveToSignalObject=off  IntegratorRTWStateStorageClass=Auto  FilterContinuousStateAttributes=''  FilterStateMustResolveToSignalObject=off  FilterRTWStateStorageClass=Auto  ParallelPVariant=InternalParameters  IdealPVariant=Disabled  IVariant=Disabled  DVariant=InternalParameters  IntegratorVariant=Disabled  SatVariant=Enabled  AWVariant=Disabled  PCopyVariant=Disabled  TRVariant=Disabled  FdbkBlocksVariant=Forward  IdealPFdbkVariant=Disabled  SatFdbkVariant=Disabled  DerivativeFilterVariant=Differentiator  NVariant=Passthrough  NCopyVariant=Disabled_SignalSpec  FilterICVariant=InternalICsDifferentiator  IntegratorICVariant=Disabled  ExternalResetVariant=Disabled  TRSumVariant=Passthrough  SumFdbkVariant=Disabled  SumVariant=Sum_PD  TsampFilterVariant=InternalTs  TsampNgainVariant=Passthrough  TsampIntegralVariant=Disabled_SignalSpec  ExternalSaturationOutDataTypeStr=Inherit: Same as second input  DerivativeSourceVariant=ErrorSignal
  Quaternions to Rotation Angles : sharedtransform/Quaternions to Rotation Angles  rotationOrder=XYZ  aMode=aMode
  Selector : Selector  InputPortWidth=3  IndexOptions=Index vector (dialog)  Indices=[3]  OutputSizes=1
  T : Outport
  wires:
  q/1 -> Quaternions to Rotation Angles/1
  Quaternions to Rotation Angles/1 -> Selector/1
  Demo Controller/1 -> T/1
  Selector/1 -> Demo Controller/1

== system SolarSailOld/Reaction Wheel ==
  Torque Vector : Inport
  Constant : Constant  Value=10^-3
  Constant7 : Constant  Value=[0;0]
  Torque Limiter : MATLAB Function  TreatAsAtomicUnit=on
  Vector Concatenate : Concatenate
  RW Torque Vector : Outport
  wires:
  Vector Concatenate/1 -> RW Torque Vector/1
  Constant7/1 -> Vector Concatenate/1
  Constant/1 -> Torque Limiter/2(limit)
  Torque Limiter/1(T) -> Vector Concatenate/2
  Torque Vector/1 -> Torque Limiter/1(desired_T)

== system SolarSailOld/SRP Force Model ==
  Sun Angle : Inport
  Attitude : Inport  Port=2
  BusElementIn : Inport  Port=3  PortName=Constants  Element=SRP
  BusElementIn1 : Inport  Port=3  PortName=Constants  Element=Solar Sail Area
  Multiplication : Subsystem
  Normal : Constant  Value=[0;0;1]
  Product : Product  Multiplication=Matrix(*)
  Product1 : Product
  Quat2RotMat : MATLAB Function  TreatAsAtomicUnit=on
  SRP Force : Outport
  wires:
  Sun Angle/1 -> Multiplication/2(Sun Angle)
  Attitude/1 -> Quat2RotMat/1(quat)
  Product/1 -> Product1/2
  Quat2RotMat/1(rotm) -> Product/1
  Normal/1 -> Product/2
  Multiplication/1(SRP Force) -> Product1/1
  Product1/1 -> SRP Force/1
  BusElementIn/1 -> Multiplication/1(SRP)
  BusElementIn1/1 -> Multiplication/3(Area)

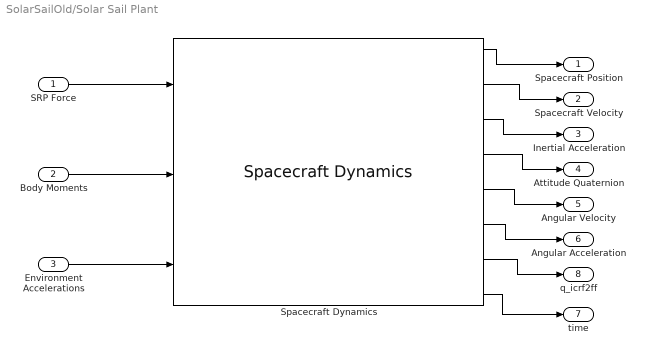
== system SolarSailOld/Solar Sail Plant ==
  SRP Force : Inport
  Body Moments : Inport  Port=2
  Environment Accelerations : Inport  Port=3
  Spacecraft Dynamics : SpacecraftDynamics  accelIn=on  outputAccel=on  startDate=juliandate(2024, 7, 11, 2, 0, 0)  mass=3.0  inertia=[1,0,0;0,1,0;0,0,1]  semiMajorAxis=7078140  eccentricity=0.001  inclination=98.1928  raan=22  argPeriapsis=360  trueAnomaly=0  attitude=[0.719,-0.0985,-0.6633,-0.1827]  outputAngAccel=on  outputTransform=on  ephemerisModel=DE432t  srpArea=32
  Spacecraft Position : Outport
  Spacecraft Velocity : Outport  Port=2
  Inertial Acceleration : Outport  Port=3
  Attitude Quaternion : Outport  Port=4
  Angular Velocity : Outport  Port=5
  Angular Acceleration : Outport  Port=6
  time : Outport  Port=7
  q_icrf2ff : Outport  Port=8
  wires:
  Environment Accelerations/1 -> Spacecraft Dynamics/3
  Body Moments/1 -> Spacecraft Dynamics/2
  SRP Force/1 -> Spacecraft Dynamics/1
  Spacecraft Dynamics/1 -> Spacecraft Position/1
  Spacecraft Dynamics/2 -> Spacecraft Velocity/1
  Spacecraft Dynamics/3 -> Inertial Acceleration/1
  Spacecraft Dynamics/4 -> Attitude Quaternion/1
  Spacecraft Dynamics/5 -> Angular Velocity/1
  Spacecraft Dynamics/6 -> Angular Acceleration/1
  Spacecraft Dynamics/8 -> time/1
  Spacecraft Dynamics/7 -> q_icrf2ff/1

== system SolarSailOld/Solar Sail Plant1 ==
  SRP Force : Inport
  Body Moments : Inport  Port=2
  Environment Accelerations : Inport  Port=3
  Spacecraft Dynamics : SpacecraftDynamics  accelIn=on  accelFrame=Fixed-frame  outportFrame=Fixed-frame  outputAccel=on  mass=3.0  inertia=[344.15, 0, 0; 0, 344.15, 0; 0, 0, 688.24]  semiMajorAxis=7078140  eccentricity=0.001  inclination=98.1928  raan=22  argPeriapsis=360  trueAnomaly=0  attitudeFrame=LVLH  attitude=[0.6533,-0.2706,0.2706,-0.6533]  outputAngAccel=on  ephemerisModel=DE432t  srpArea=32
  Spacecraft Position : Outport
  Spacecraft Velocity : Outport  Port=2
  Inertial Acceleration : Outport  Port=3
  Attitude Quaternion : Outport  Port=4
  Angular Velocity : Outport  Port=5
  Angular Acceleration : Outport  Port=6
  time : Outport  Port=7
  wires:
  Environment Accelerations/1 -> Spacecraft Dynamics/3
  Body Moments/1 -> Spacecraft Dynamics/2
  SRP Force/1 -> Spacecraft Dynamics/1
  Spacecraft Dynamics/1 -> Spacecraft Position/1
  Spacecraft Dynamics/2 -> Spacecraft Velocity/1
  Spacecraft Dynamics/3 -> Inertial Acceleration/1
  Spacecraft Dynamics/4 -> Attitude Quaternion/1
  Spacecraft Dynamics/5 -> Angular Velocity/1
  Spacecraft Dynamics/6 -> Angular Acceleration/1
  Spacecraft Dynamics/7 -> time/1

== system SolarSailOld/Sun Angle ==
  Attitude : Inport
  julian_date : Inport  Port=2
  Spacecraft Position : Inport  Port=3
  MATLAB Function : MATLAB Function  TreatAsAtomicUnit=on
  Math Function : Math  Operator=magnitude^2
  Normal : Constant  Value=[0;0;1]
  Product : Product  Multiplication=Matrix(*)
  Quat2RotMat : MATLAB Function  TreatAsAtomicUnit=on
  Subtract : Sum  Inputs=+-
  sun_position : MATLAB Function  TreatAsAtomicUnit=on
  Sun Angle : Outport
  wires:
  Normal/1 -> Product/2
  Quat2RotMat/1(rotm) -> Product/1
  Product/1 -> MATLAB Function/1(N_icrf)  "N_icrf"
  Attitude/1 -> Quat2RotMat/1(quat)
  Subtract/1 -> MATLAB Function/2(r_satsun)  "r_satsun"
  Spacecraft Position/1 -> Subtract/2  "r_sat"
  sun_position/1(r_sun) -> Subtract/1  "r_sun"
  julian_date/1 -> sun_position/1(julian_date)
  MATLAB Function/1(sunAngle) -> Sun Angle/1

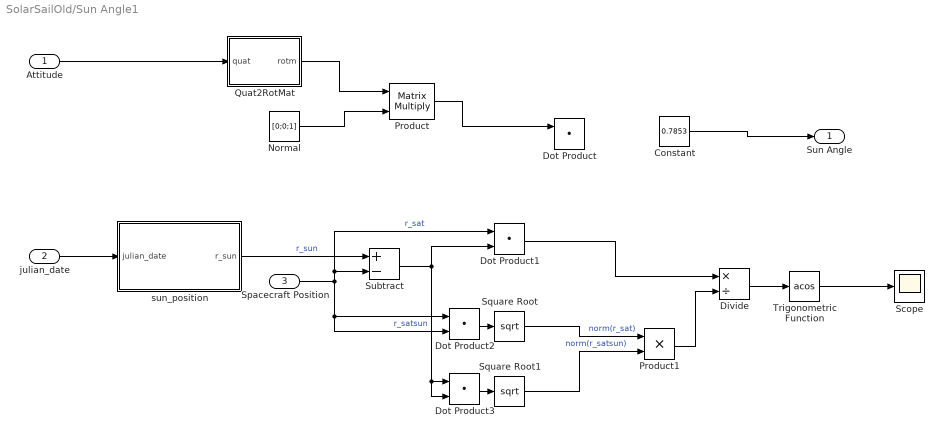
== system SolarSailOld/Sun Angle1 ==
  Attitude : Inport
  julian_date : Inport  Port=2
  Spacecraft Position : Inport  Port=3
  Constant : Constant  Value=0.7853
  Divide : Product  Inputs=*/
  Dot Product{,1..3} (4 alike) : DotProduct  OutDataTypeStr=Inherit: Inherit via internal rule
  Normal : Constant  Value=[0;0;1]
  Product : Product  Multiplication=Matrix(*)
  Product1 : Product
  Quat2RotMat : MATLAB Function  TreatAsAtomicUnit=on
  Scope : Scope
  Square Root : Sqrt
  Square Root1 : Sqrt
  Subtract : Sum  Inputs=+-
  Trigonometric Function : Trigonometry  Operator=acos
  sun_position : MATLAB Function  TreatAsAtomicUnit=on
  Sun Angle : Outport
  wires:
  julian_date/1 -> sun_position/1(julian_date)
  sun_position/1(r_sun) -> Subtract/1  "r_sun"
  Spacecraft Position/1 -> Dot Product1/1, Subtract/2, Dot Product2/2, Dot Product2/1  "r_sat"
  Subtract/1 -> Dot Product3/2, Dot Product3/1, Dot Product1/2  "r_satsun"
  Attitude/1 -> Quat2RotMat/1(quat)
  Product/1 -> Dot Product/1
  Quat2RotMat/1(rotm) -> Product/1
  Normal/1 -> Product/2
  Dot Product2/1 -> Square Root/1
  Dot Product3/1 -> Square Root1/1
  Square Root/1 -> Product1/1  "norm(r_sat)"
  Square Root1/1 -> Product1/2  "norm(r_satsun)"
  Dot Product1/1 -> Divide/1
  Product1/1 -> Divide/2
  Divide/1 -> Trigonometric Function/1
  Trigonometric Function/1 -> Scope/1
  Constant/1 -> Sun Angle/1

== system SolarSailOld/icrf2lvlh ==
  quat_icrf : Inport
  pos_icrf : Inport  Port=2
  vel_icrf : Inport  Port=3
  Direction Cosine Matrix to Quaternions : sharedtransform/Direction Cosine Matrix  to Quaternions  aMode=0  action=Warning  tolerance=eps(4)
      settings: LibrarySourceBlock=|
      | aerolibtransform2/Direction Cosine Matrix
      | to Quaternions
  MATLAB Function : MATLAB Function  TreatAsAtomicUnit=on
  Quaternion Multiplication : aerolibutil/Quaternion Multiplication
  quat_lvlh : Outport
  wires:
  pos_icrf/1 -> MATLAB Function/1(pos)
  vel_icrf/1 -> MATLAB Function/2(vel)
  MATLAB Function/1(DCM) -> Direction Cosine Matrix to Quaternions/1
  quat_icrf/1 -> Quaternion Multiplication/2
  Direction Cosine Matrix to Quaternions/1 -> Quaternion Multiplication/1
  Quaternion Multiplication/1 -> quat_lvlh/1

== system SolarSailOld/pos2radius ==
  pos : Inport
  Dot Product : DotProduct  OutDataTypeStr=Inherit: Inherit via internal rule
  Square Root : Sqrt
  Radius : Outport
  wires:
  pos/1 -> Dot Product/2, Dot Product/1
  Dot Product/1 -> Square Root/1
  Square Root/1 -> Radius/1  "Radius"

== system SolarSailOld/CubeSat Animation/Antenna Position to VRML ==
  x : Inport
  ECEF to VRML : Subsystem
  Length Conversion : aerolibconvert2/Length Conversion  IU=m  OU=km
  km to VRML units : Gain  Gain=1/1000
  xVRML : Outport  VectorParamsAs1DForOutWhenUnconnected=off
  wires:
  Length Conversion/1 -> km to VRML units/1
  km to VRML units/1 -> ECEF to VRML/1(M)
  x/1 -> Length Conversion/1
  ECEF to VRML/1(VR) -> xVRML/1

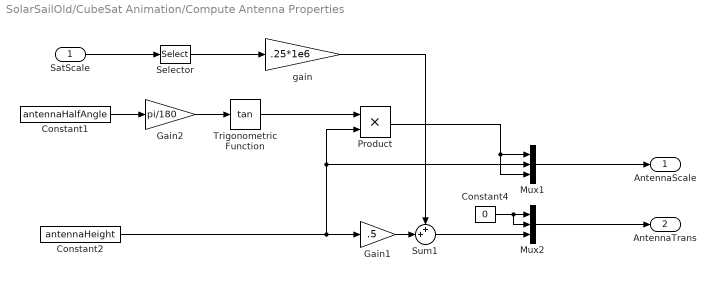
== system SolarSailOld/CubeSat Animation/Compute Antenna Properties ==
  SatScale : Inport
  Constant1 : Constant  Value=antennaHalfAngle
  Constant2 : Constant  Value=antennaHeight
  Constant4 : Constant  Value=0
  Gain1 : Gain  Gain=.5
  Gain2 : Gain  Gain=pi/180
  Mux1 : Mux  Inputs=3
  Mux2 : Mux  Inputs=3
  Product : Product
  Selector : Selector  InputPortWidth=3  IndexOptions=Index vector (dialog)  Indices=1  OutputSizes=1
  Sum1 : Sum  Inputs=++|
  Trigonometric Function : Trigonometry  Operator=tan
  gain : Gain  Gain=.25*1e6
  AntennaScale : Outport  VectorParamsAs1DForOutWhenUnconnected=off
  AntennaTrans : Outport  Port=2  VectorParamsAs1DForOutWhenUnconnected=off
  wires:
  Gain2/1 -> Trigonometric Function/1
  Constant4/1 -> Mux2/1, Mux2/2
  Sum1/1 -> Mux2/3
  Constant2/1 -> Gain1/1, Mux1/2, Product/2
  gain/1 -> Sum1/1
  Constant1/1 -> Gain2/1
  Product/1 -> Mux1/3, Mux1/1
  Gain1/1 -> Sum1/2
  Trigonometric Function/1 -> Product/1
  Mux2/1 -> AntennaTrans/1
  Mux1/1 -> AntennaScale/1
  SatScale/1 -> Selector/1
  Selector/1 -> gain/1

== system SolarSailOld/CubeSat Animation/Compute Earth Rotation Rate ==
  EarthRot : Inport
  Constant : Constant  Value=0
  Constant1 : Constant  Value=0
  Euler Angles to Quaternions : aerolibobsolete/Euler Angles to Quaternions
  Quaternion to VRML : Subsystem
  Sum : Sum  Inputs=|++
  Unit Delay : UnitDelay  SampleTime=-1  HasFrameUpgradeWarning=on
  Vector Concatenate : Concatenate  NumInputs=3
  VRMLRot : Outport  VectorParamsAs1DForOutWhenUnconnected=off
  wires:
  Quaternion to VRML/1(AxisAngle) -> VRMLRot/1
  Euler Angles to Quaternions/1 -> Quaternion to VRML/1(q)
  Vector Concatenate/1 -> Euler Angles to Quaternions/1
  Constant1/1 -> Vector Concatenate/2
  Constant/1 -> Vector Concatenate/1
  Sum/1 -> Unit Delay/1, Vector Concatenate/3
  Unit Delay/1 -> Sum/2
  EarthRot/1 -> Sum/1

== system SolarSailOld/CubeSat Animation/Compute Umbra Translation ==
  I : Inport
  Add : Sum
  ConeHalfLength : Gain  Gain=692
  InvertSunPosECEF : Gain  Gain=-1
  unitVec : Subsystem
  O : Outport  VectorParamsAs1DForOutWhenUnconnected=off
  wires:
  ConeHalfLength/1 -> Add/2
  I/1 -> InvertSunPosECEF/1
  Add/1 -> O/1
  InvertSunPosECEF/1 -> unitVec/1(I), Add/1
  unitVec/1(O) -> ConeHalfLength/1

== system SolarSailOld/CubeSat Animation/Quaternion to VRML ==
  q : Inport
  Demux : Demux
  "Flip 180 deg, rotate 90" : Constant  Value=[0 -.7071 .7071 0]
  Gain : Gain  Gain=2
  Mux : Mux
  Quaternion Multiplication : aerolibutil/Quaternion Multiplication
  Selector : Selector  InputPortWidth=4  IndexOptions=Index vector (dialog)  Indices=[3 4 2 1]  OutputSizes=1
  Trigonometric Function : Trigonometry  Operator=acos
  axis_angle : Outport  VectorParamsAs1DForOutWhenUnconnected=off
  wires:
  Demux/4 -> Mux/4
  Demux/3 -> Mux/3
  Demux/2 -> Mux/2
  Gain/1 -> Mux/1
  Selector/1 -> axis_angle/1
  q/1 -> Quaternion Multiplication/1
  Mux/1 -> Selector/1
  Trigonometric Function/1 -> Gain/1
  Demux/1 -> Trigonometric Function/1
  "Flip 180 deg, rotate 90"/1 -> Quaternion Multiplication/2
  Quaternion Multiplication/1 -> Demux/1

== system SolarSailOld/CubeSat Animation/Quaternion to VRML1 ==
  q : Inport
  Demux : Demux
  "Flip 180 deg, rotate 90" : Constant  Value=[0 -0.7071 0.7071 0]
  Gain : Gain  Gain=2
  Mux : Mux
  Quaternion Multiplication : aerolibutil/Quaternion Multiplication
  Selector : Selector  InputPortWidth=4  IndexOptions=Index vector (dialog)  Indices=[3 4 2 1]  OutputSizes=1
  Trigonometric Function : Trigonometry  Operator=acos
  axis_angle : Outport  VectorParamsAs1DForOutWhenUnconnected=off
  wires:
  Demux/4 -> Mux/4
  Demux/3 -> Mux/3
  Demux/2 -> Mux/2
  Gain/1 -> Mux/1
  Selector/1 -> axis_angle/1
  Mux/1 -> Selector/1
  Trigonometric Function/1 -> Gain/1
  Demux/1 -> Trigonometric Function/1
  "Flip 180 deg, rotate 90"/1 -> Quaternion Multiplication/2
  q/1 -> Quaternion Multiplication/1
  Quaternion Multiplication/1 -> Demux/1

== system SolarSailOld/CubeSat Animation/Radar on//off ==
  NavMode : Inport
  Add : Sum  Inputs=-+
  Compare To Constant : simulink/Logic and Bit Operations/Compare To Constant  relop===  const=1  OutDataTypeStr=boolean  ZeroCross=off
  Constant : Constant
  Data Type Conversion : DataTypeConversion  OutDataTypeStr=double  SaturateOnIntegerOverflow=off  RndMeth=Floor
  Gain : Gain  Gain=0.6
  Radar : Outport  VectorParamsAs1DForOutWhenUnconnected=off
  wires:
  NavMode/1 -> Compare To Constant/1
  Compare To Constant/1 -> Data Type Conversion/1
  Data Type Conversion/1 -> Gain/1
  Gain/1 -> Add/1
  Constant/1 -> Add/2
  Add/1 -> Radar/1

== system SolarSailOld/CubeSat Animation/Sat Position to VRML ==
  x : Inport
  ECEF to VRML : Subsystem
  Length Conversion : aerolibconvert2/Length Conversion  IU=m  OU=km
  km to VRML units : Gain  Gain=1/1000
  xVRML : Outport  VectorParamsAs1DForOutWhenUnconnected=off
  wires:
  ECEF to VRML/1(VR) -> xVRML/1
  x/1 -> Length Conversion/1
  km to VRML units/1 -> ECEF to VRML/1(M)
  Length Conversion/1 -> km to VRML units/1

== system SolarSailOld/CubeSat Animation/Satellite Model Scaling ==
  Constant : Constant  Value=cubesatSize
  Mux : Mux  Inputs=3
  ScaleModelToVRML : Gain  Gain=1/.3e6
  Out1 : Outport  VectorParamsAs1DForOutWhenUnconnected=off
  wires:
  ScaleModelToVRML/1 -> Mux/3, Mux/1, Mux/2
  Constant/1 -> ScaleModelToVRML/1
  Mux/1 -> Out1/1

== system SolarSailOld/CubeSat Animation/Sun Position to VRML ==
  x : Inport
  ECEF to VRML : Subsystem
  Length Conversion : aerolibconvert2/Length Conversion  IU=m  OU=km
  km to VRML units : Gain  Gain=1/1000
  xVRML : Outport  VectorParamsAs1DForOutWhenUnconnected=off
  wires:
  ECEF to VRML/1(VR) -> xVRML/1
  x/1 -> Length Conversion/1
  km to VRML units/1 -> ECEF to VRML/1(M)
  Length Conversion/1 -> km to VRML units/1

== system SolarSailOld/RCD Converter/If Action Subsystem ==
  Action Port : ActionPort  InitializeStates=reset  ActionPortLabel=elseif(u1 < -u2)
  Constant : Constant  Value=0
  Constant1 : Constant
  RCD2 : Outport
  RCD4 : Outport  Port=2
  wires:
  Constant/1 -> RCD2/1
  Constant1/1 -> RCD4/1

== system SolarSailOld/RCD Converter/If Action Subsystem1 ==
  Action Port : ActionPort  InitializeStates=reset  ActionPortLabel=if(u1 > u2)
  Constant : Constant
  Constant1 : Constant  Value=0
  RCD1 : Outport
  RCD3 : Outport  Port=2
  wires:
  Constant1/1 -> RCD1/1
  Constant/1 -> RCD3/1

== system SolarSailOld/RCD Converter/If Action Subsystem2 ==
  Action Port : ActionPort  InitializeStates=reset  ActionPortLabel=elseif(u1 < -u2)
  Constant : Constant
  Constant1 : Constant  Value=0
  RCD1 : Outport
  RCD3 : Outport  Port=2
  wires:
  Constant/1 -> RCD1/1
  Constant1/1 -> RCD3/1

== system SolarSailOld/RCD Converter/If Action Subsystem3 ==
  Action Port : ActionPort  InitializeStates=reset  ActionPortLabel=if(u1 > u2)
  Constant : Constant
  Constant1 : Constant  Value=0
  RCD2 : Outport
  RCD4 : Outport  Port=2
  wires:
  Constant/1 -> RCD2/1
  Constant1/1 -> RCD4/1

== system SolarSailOld/RCD Converter/If Action Subsystem4 ==
  Action Port : ActionPort  ActionPortLabel=else
  Constant : Constant  Value=0
  Constant1 : Constant  Value=0
  RCD2 : Outport
  RCD4 : Outport  Port=2
  wires:
  Constant1/1 -> RCD4/1
  Constant/1 -> RCD2/1

== system SolarSailOld/RCD Converter/If Action Subsystem5 ==
  Action Port : ActionPort  ActionPortLabel=else
  Constant : Constant  Value=0
  Constant1 : Constant  Value=0
  RCD1 : Outport
  RCD3 : Outport  Port=2
  wires:
  Constant1/1 -> RCD3/1
  Constant/1 -> RCD1/1

== system SolarSailOld/RCD Diffusive Force/F_normal ==
  SRP : Inport
  area : Inport  Port=2
  sun anlge : Inport  Port=3
  Cos : Trigonometry  Operator=cos
  Gain : Gain  Gain=2/3
  Product1 : Product  Inputs=3
  F_normal : Outport
  wires:
  Cos/1 -> Product1/3
  Product1/1 -> Gain/1
  SRP/1 -> Product1/1
  area/1 -> Product1/2  "area"
  sun anlge/1 -> Cos/1
  Gain/1 -> F_normal/1

== system SolarSailOld/RCD Diffusive Force/F_sun ==
  SRP : Inport
  area : Inport  Port=2
  sun anlge : Inport  Port=3
  Cos : Trigonometry  Operator=cos
  Product1 : Product  Inputs=3
  F_sun : Outport
  wires:
  Cos/1 -> Product1/3
  Product1/1 -> F_sun/1
  sun anlge/1 -> Cos/1
  area/1 -> Product1/2  "area"
  SRP/1 -> Product1/1

== system SolarSailOld/RCD Diffusive Force1/F_normal ==
  SRP : Inport
  area : Inport  Port=2
  sun anlge : Inport  Port=3
  Cos : Trigonometry  Operator=cos
  Gain : Gain  Gain=2/3
  Product1 : Product  Inputs=3
  F_normal : Outport
  wires:
  Cos/1 -> Product1/3
  Product1/1 -> Gain/1
  SRP/1 -> Product1/1
  area/1 -> Product1/2  "area"
  sun anlge/1 -> Cos/1
  Gain/1 -> F_normal/1

== system SolarSailOld/RCD Diffusive Force1/F_sun ==
  SRP : Inport
  area : Inport  Port=2
  sun anlge : Inport  Port=3
  Cos : Trigonometry  Operator=cos
  Product1 : Product  Inputs=3
  F_sun : Outport
  wires:
  Cos/1 -> Product1/3
  Product1/1 -> F_sun/1
  sun anlge/1 -> Cos/1
  area/1 -> Product1/2  "area"
  SRP/1 -> Product1/1

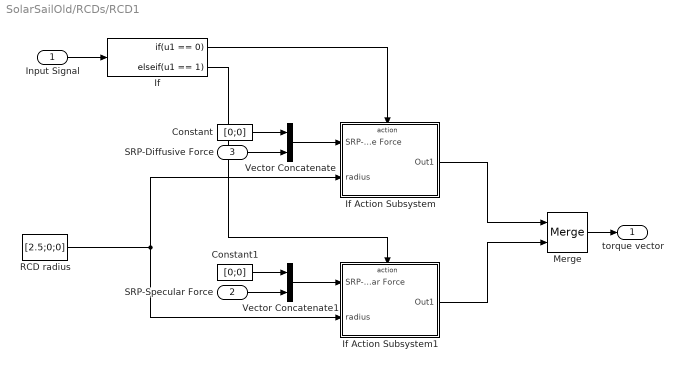
== system SolarSailOld/RCDs/RCD1 ==
  Input Signal : Inport
  SRP-Specular Force : Inport  Port=2
  SRP-Diffusive Force : Inport  Port=3
  Constant : Constant  Value=[0;0]
  Constant1 : Constant  Value=[0;0]
  If : If  IfExpression=u1 == 0  ElseIfExpressions=u1 == 1  ShowElse=off
  If Action Subsystem : Subsystem  TreatAsAtomicUnit=on
  If Action Subsystem1 : Subsystem  TreatAsAtomicUnit=on
  Merge : Merge
  RCD radius : Constant  Value=[2.5;0;0]
  Vector Concatenate : Concatenate
  Vector Concatenate1 : Concatenate
  torque vector : Outport
  wires:
  Input Signal/1 -> If/1
  If/1 -> If Action Subsystem/Action
  Merge/1 -> torque vector/1
  If Action Subsystem/1(Out1) -> Merge/1
  If/2 -> If Action Subsystem1/Action
  If Action Subsystem1/1(Out1) -> Merge/2
  RCD radius/1 -> If Action Subsystem/2(radius), If Action Subsystem1/2(radius)
  Vector Concatenate/1 -> If Action Subsystem/1(SRP-Diffusive Force)
  Constant/1 -> Vector Concatenate/1
  SRP-Diffusive Force/1 -> Vector Concatenate/2
  SRP-Specular Force/1 -> Vector Concatenate1/2
  Constant1/1 -> Vector Concatenate1/1
  Vector Concatenate1/1 -> If Action Subsystem1/1(SRP-Specular Force)
